simulink model "14_bus"  (R2024a)
settings: Solver=VariableStepAuto  StartTime=0.0  StopTime=1  RelTol=1e-3
undefined symbols (not defined in the file): D1, Delta
libraries: spsRMSLib x186, simulink_extras x171, spsThreePhaseVIMeasurementLib x94, spsThreePhaseBreakerLib x62, spsThreePhaseSeriesRLCBranchLib x20, spsThreePhaseSeriesRLCLoadLib x12, spsThreePhaseSourceLib x5, spsLoadFlowBusLib x5, spsStairGeneratorLib x5, spsThreePhaseTransformerTwoWindingsLib x5, spsThreePhaseFaultLib x5, sps_lib x1
(part 2 of 6)

== system 14_bus/BUS_3 ==
  Bus-3 : spsThreePhaseVIMeasurementLib/Three-Phase V-I Measurement  VoltageMeasurement=phase-to-ground  SetLabelV=on  LabelV=VB3  Vpu=off  VpuLL=off  CurrentMeasurement=yes  SetLabelI=on  LabelI=IB3  Ipu=off  Pbase=100e6  Vbase=0.95  OutputType=Complex  PhasorSimulation=off  PSBequivalent=0
  Bus3 : spsThreePhaseVIMeasurementLib/Three-Phase V-I Measurement  VoltageMeasurement=phase-to-ground  SetLabelV=on  LabelV=VB_3  Vpu=off  VpuLL=off  CurrentMeasurement=yes  SetLabelI=on  LabelI=IB_3  Ipu=off  Pbase=100e6  Vbase=0.95  OutputType=Complex  PhasorSimulation=off  PSBequivalent=0
  Bus_3 : spsThreePhaseVIMeasurementLib/Three-Phase V-I Measurement  VoltageMeasurement=phase-to-ground  SetLabelV=on  LabelV=V_B3  Vpu=off  VpuLL=off  CurrentMeasurement=yes  SetLabelI=on  LabelI=I_B3  Ipu=off  Pbase=100e6  Vbase=0.95  OutputType=Complex  PhasorSimulation=off  PSBequivalent=0
  C : PMIOPort  Side=Left
  B : PMIOPort  Port=2  Side=Left
  C1 : PMIOPort  Port=3  Side=Left
  c : PMIOPort  Port=4  Side=Right
  b : PMIOPort  Port=5  Side=Right
  a : PMIOPort  Port=6  Side=Right
  a1 : PMIOPort  Port=7  Side=Right
  b1 : PMIOPort  Port=8  Side=Right
  c1 : PMIOPort  Port=9  Side=Right
  a2 : PMIOPort  Port=10  Side=Right
  b2 : PMIOPort  Port=11  Side=Right
  c2 : PMIOPort  Port=12  Side=Right
  connections:
  b/RConn1 -- Bus-3/RConn2
  Bus_3/LConn3 -- Bus3/LConn1 -- C/RConn1 -- Bus-3/LConn3
  a/RConn1 -- Bus-3/RConn1
  c1/RConn1 -- Bus3/RConn3
  c/RConn1 -- Bus-3/RConn3
  Bus-3/LConn2 -- B/RConn1 -- Bus3/LConn2 -- Bus_3/LConn2
  Bus_3/LConn1 -- C1/RConn1 -- Bus-3/LConn1 -- Bus3/LConn3
  c2/RConn1 -- Bus_3/RConn3
  a1/RConn1 -- Bus3/RConn1
  b2/RConn1 -- Bus_3/RConn2
  b1/RConn1 -- Bus3/RConn2
  a2/RConn1 -- Bus_3/RConn1

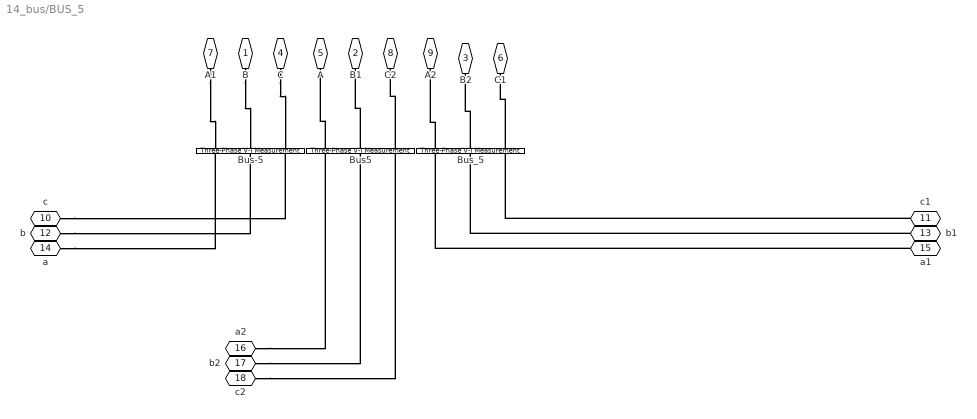
== system 14_bus/BUS_5 ==
  Bus-5 : spsThreePhaseVIMeasurementLib/Three-Phase V-I Measurement  VoltageMeasurement=phase-to-ground  SetLabelV=on  LabelV=VB5  Vpu=off  VpuLL=off  CurrentMeasurement=yes  SetLabelI=on  LabelI=IB5  Ipu=off  Pbase=100e6  Vbase=0.95  OutputType=Complex  PhasorSimulation=off  PSBequivalent=0
  Bus5 : spsThreePhaseVIMeasurementLib/Three-Phase V-I Measurement  VoltageMeasurement=phase-to-ground  SetLabelV=on  LabelV=VB_5  Vpu=off  VpuLL=off  CurrentMeasurement=yes  SetLabelI=on  LabelI=IB_5  Ipu=off  Pbase=100e6  Vbase=0.95  OutputType=Complex  PhasorSimulation=off  PSBequivalent=0
  Bus_5 : spsThreePhaseVIMeasurementLib/Three-Phase V-I Measurement  VoltageMeasurement=phase-to-ground  SetLabelV=on  LabelV=V_B5  Vpu=off  VpuLL=off  CurrentMeasurement=yes  SetLabelI=on  LabelI=I_B5  Ipu=off  Pbase=100e6  Vbase=0.95  OutputType=Complex  PhasorSimulation=off  PSBequivalent=0
  B : PMIOPort  Side=Left
  B1 : PMIOPort  Port=2  Side=Left
  B2 : PMIOPort  Port=3  Side=Left
  C : PMIOPort  Port=4  Side=Left
  A : PMIOPort  Port=5  Side=Left
  C1 : PMIOPort  Port=6  Side=Left
  A1 : PMIOPort  Port=7  Side=Left
  C2 : PMIOPort  Port=8  Side=Left
  A2 : PMIOPort  Port=9  Side=Left
  c : PMIOPort  Port=10  Side=Right
  c1 : PMIOPort  Port=11  Side=Right
  b : PMIOPort  Port=12  Side=Right
  b1 : PMIOPort  Port=13  Side=Right
  a : PMIOPort  Port=14  Side=Right
  a1 : PMIOPort  Port=15  Side=Right
  a2 : PMIOPort  Port=16  Side=Right
  b2 : PMIOPort  Port=17  Side=Right
  c2 : PMIOPort  Port=18  Side=Right
  connections:
  b/RConn1 -- Bus-5/RConn2
  c2/RConn1 -- Bus5/RConn3
  Bus5/LConn1 -- A/RConn1
  C/RConn1 -- Bus-5/LConn3
  Bus_5/LConn1 -- A2/RConn1
  c1/RConn1 -- Bus_5/RConn3
  B/RConn1 -- Bus-5/LConn2
  a1/RConn1 -- Bus_5/RConn1
  a2/RConn1 -- Bus5/RConn1
  Bus5/LConn2 -- B1/RConn1
  Bus_5/LConn2 -- B2/RConn1
  b1/RConn1 -- Bus_5/RConn2
  b2/RConn1 -- Bus5/RConn2
  c/RConn1 -- Bus-5/RConn3
  Bus5/LConn3 -- C2/RConn1
  A1/RConn1 -- Bus-5/LConn1
  Bus_5/LConn3 -- C1/RConn1
  a/RConn1 -- Bus-5/RConn1

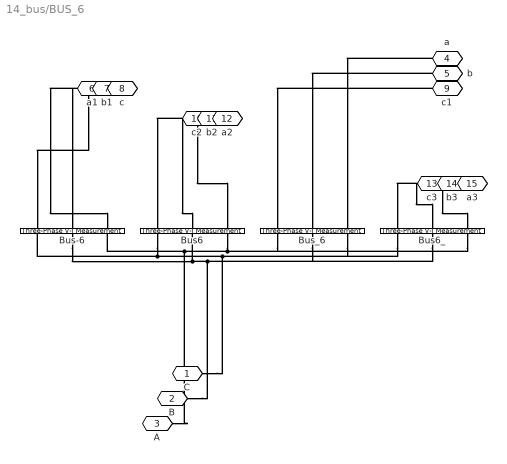
== system 14_bus/BUS_6 ==
  Bus-6 : spsThreePhaseVIMeasurementLib/Three-Phase V-I Measurement  VoltageMeasurement=phase-to-ground  SetLabelV=on  LabelV=VB6  Vpu=off  VpuLL=off  CurrentMeasurement=yes  SetLabelI=on  LabelI=IB6  Ipu=off  Pbase=100e6  Vbase=0.95  OutputType=Complex  PhasorSimulation=off  PSBequivalent=0
  Bus6 : spsThreePhaseVIMeasurementLib/Three-Phase V-I Measurement  VoltageMeasurement=phase-to-ground  SetLabelV=on  LabelV=VB_6  Vpu=off  VpuLL=off  CurrentMeasurement=yes  SetLabelI=on  LabelI=IB_6  Ipu=off  Pbase=100e6  Vbase=0.95  OutputType=Complex  PhasorSimulation=off  PSBequivalent=0
  Bus6_ : spsThreePhaseVIMeasurementLib/Three-Phase V-I Measurement  VoltageMeasurement=phase-to-ground  SetLabelV=on  LabelV=VB6_  Vpu=off  VpuLL=off  CurrentMeasurement=yes  SetLabelI=on  LabelI=IB6_  Ipu=off  Pbase=100e6  Vbase=0.95  OutputType=Complex  PhasorSimulation=off  PSBequivalent=0
  Bus_6 : spsThreePhaseVIMeasurementLib/Three-Phase V-I Measurement  VoltageMeasurement=phase-to-ground  SetLabelV=on  LabelV=V_B6  Vpu=off  VpuLL=off  CurrentMeasurement=yes  SetLabelI=on  LabelI=I_B6  Ipu=off  Pbase=100e6  Vbase=0.95  OutputType=Complex  PhasorSimulation=off  PSBequivalent=0
  C : PMIOPort  Side=Left
  B : PMIOPort  Port=2  Side=Left
  A : PMIOPort  Port=3  Side=Left
  a : PMIOPort  Port=4  Side=Right
  b : PMIOPort  Port=5  Side=Right
  a1 : PMIOPort  Port=6  Side=Right
  b1 : PMIOPort  Port=7  Side=Right
  c : PMIOPort  Port=8  Side=Right
  c1 : PMIOPort  Port=9  Side=Right
  c2 : PMIOPort  Port=10  Side=Right
  b2 : PMIOPort  Port=11  Side=Right
  a2 : PMIOPort  Port=12  Side=Right
  c3 : PMIOPort  Port=13  Side=Right
  b3 : PMIOPort  Port=14  Side=Right
  a3 : PMIOPort  Port=15  Side=Right
  connections:
  Bus6_/LConn1 -- Bus_6/LConn3 -- Bus6/LConn1 -- A/RConn1 -- Bus-6/LConn1
  b/RConn1 -- Bus_6/RConn2
  Bus6_/LConn3 -- Bus_6/LConn1 -- C/RConn1 -- Bus6/LConn3 -- Bus-6/LConn3
  c/RConn1 -- Bus-6/RConn3
  Bus6_/LConn2 -- Bus_6/LConn2 -- B/RConn1 -- Bus-6/LConn2 -- Bus6/LConn2
  a/RConn1 -- Bus_6/RConn1
  b1/RConn1 -- Bus-6/RConn2
  a3/RConn1 -- Bus6_/RConn1
  c1/RConn1 -- Bus_6/RConn3
  c3/RConn1 -- Bus6_/RConn3
  b3/RConn1 -- Bus6_/RConn2
  c2/RConn1 -- Bus6/RConn3
  a1/RConn1 -- Bus-6/RConn1
  a2/RConn1 -- Bus6/RConn1
  b2/RConn1 -- Bus6/RConn2

== system 14_bus/BUS_7 ==
  Bus-7 : spsThreePhaseVIMeasurementLib/Three-Phase V-I Measurement  VoltageMeasurement=phase-to-ground  SetLabelV=on  LabelV=VB7  Vpu=off  VpuLL=off  CurrentMeasurement=yes  SetLabelI=on  LabelI=IB7  Ipu=off  Pbase=100e6  Vbase=0.95  OutputType=Complex  PhasorSimulation=off  PSBequivalent=0
  Bus7 : spsThreePhaseVIMeasurementLib/Three-Phase V-I Measurement  VoltageMeasurement=phase-to-ground  SetLabelV=on  LabelV=VB_7  Vpu=off  VpuLL=off  CurrentMeasurement=yes  SetLabelI=on  LabelI=IB_7  Ipu=off  Pbase=100e6  Vbase=0.95  OutputType=Complex  PhasorSimulation=off  PSBequivalent=0
  a : PMIOPort  Side=Right
  b : PMIOPort  Port=2  Side=Right
  c : PMIOPort  Port=3  Side=Right
  a1 : PMIOPort  Port=4  Side=Right
  b1 : PMIOPort  Port=5  Side=Right
  c1 : PMIOPort  Port=6  Side=Right
  C : PMIOPort  Port=7  Side=Left
  B : PMIOPort  Port=8  Side=Left
  C1 : PMIOPort  Port=9  Side=Left
  connections:
  Bus7/LConn2 -- B/RConn1 -- Bus-7/LConn2
  Bus-7/LConn1 -- C/RConn1 -- Bus7/LConn3
  a1/RConn1 -- Bus7/RConn1
  Bus7/LConn1 -- Bus-7/LConn3 -- C1/RConn1
  b/RConn1 -- Bus-7/RConn2
  a/RConn1 -- Bus-7/RConn1
  b1/RConn1 -- Bus7/RConn2
  c1/RConn1 -- Bus7/RConn3
  c/RConn1 -- Bus-7/RConn3

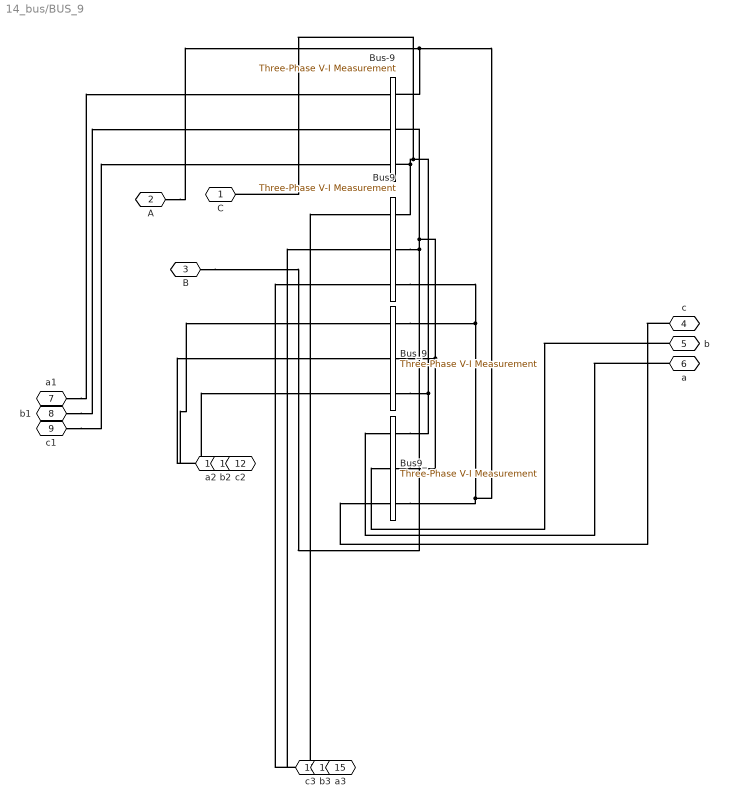
== system 14_bus/BUS_9 ==
  Bus-9 : spsThreePhaseVIMeasurementLib/Three-Phase V-I Measurement  VoltageMeasurement=phase-to-ground  SetLabelV=on  LabelV=VB9  Vpu=off  VpuLL=off  CurrentMeasurement=yes  SetLabelI=on  LabelI=IB9  Ipu=off  Pbase=100e6  Vbase=0.95  OutputType=Complex  PhasorSimulation=off  PSBequivalent=0
  Bus9 : spsThreePhaseVIMeasurementLib/Three-Phase V-I Measurement  VoltageMeasurement=phase-to-ground  SetLabelV=on  LabelV=VB_9  Vpu=off  VpuLL=off  CurrentMeasurement=yes  SetLabelI=on  LabelI=IB_9  Ipu=off  Pbase=100e6  Vbase=0.95  OutputType=Complex  PhasorSimulation=off  PSBequivalent=0
  Bus9_ : spsThreePhaseVIMeasurementLib/Three-Phase V-I Measurement  VoltageMeasurement=phase-to-ground  SetLabelV=on  LabelV=VB9_  Vpu=off  VpuLL=off  CurrentMeasurement=yes  SetLabelI=on  LabelI=IB9_  Ipu=off  Pbase=100e6  Vbase=0.95  OutputType=Complex  PhasorSimulation=off  PSBequivalent=0
  Bus_9 : spsThreePhaseVIMeasurementLib/Three-Phase V-I Measurement  VoltageMeasurement=phase-to-ground  SetLabelV=on  LabelV=V_B9  Vpu=off  VpuLL=off  CurrentMeasurement=yes  SetLabelI=on  LabelI=I_B9  Ipu=off  Pbase=100e6  Vbase=0.95  OutputType=Complex  PhasorSimulation=off  PSBequivalent=0
  C : PMIOPort  Side=Left
  A : PMIOPort  Port=2  Side=Left
  B : PMIOPort  Port=3  Side=Left
  c : PMIOPort  Port=4  Side=Right
  b : PMIOPort  Port=5  Side=Right
  a : PMIOPort  Port=6  Side=Right
  a1 : PMIOPort  Port=7  Side=Right
  b1 : PMIOPort  Port=8  Side=Right
  c1 : PMIOPort  Port=9  Side=Right
  a2 : PMIOPort  Port=10  Side=Right
  b2 : PMIOPort  Port=11  Side=Right
  c2 : PMIOPort  Port=12  Side=Right
  c3 : PMIOPort  Port=13  Side=Right
  b3 : PMIOPort  Port=14  Side=Right
  a3 : PMIOPort  Port=15  Side=Right
  connections:
  Bus9_/LConn1 -- Bus_9/LConn3 -- Bus9/LConn1 -- Bus-9/LConn3 -- C/RConn1
  A/RConn1 -- Bus-9/LConn1 -- Bus9_/LConn3 -- Bus9/LConn3 -- Bus_9/LConn1
  c/RConn1 -- Bus9_/RConn3
  B/RConn1 -- Bus9_/LConn2 -- Bus_9/LConn2 -- Bus-9/LConn2 -- Bus9/LConn2
  a3/RConn1 -- Bus9/RConn1
  c1/RConn1 -- Bus-9/RConn3
  b1/RConn1 -- Bus-9/RConn2
  c2/RConn1 -- Bus_9/RConn3
  a/RConn1 -- Bus9_/RConn1
  b2/RConn1 -- Bus_9/RConn2
  b/RConn1 -- Bus9_/RConn2
  b3/RConn1 -- Bus9/RConn2
  a2/RConn1 -- Bus_9/RConn1
  a1/RConn1 -- Bus-9/RConn1
  c3/RConn1 -- Bus9/RConn3

== system 14_bus/Subsystem1 ==
  Subsystem1 : Subsystem
  Three-Phase Breaker26 : spsThreePhaseBreakerLib/Three-Phase Breaker  InitialState=closed  SwitchA=on  SwitchB=on  SwitchC=on  SwitchTimes="[1/60  5/60]"  External=on  BreakerResistance=0.01  SnubberResistance=1e6  SnubberCapacitance=inf  Measurements=None
  VI13 : spsThreePhaseVIMeasurementLib/Three-Phase V-I Measurement  VoltageMeasurement=no  SetLabelV=off  LabelV=Vabc  Vpu=off  VpuLL=off  CurrentMeasurement=yes  SetLabelI=on  LabelI=I87  Ipu=off  Pbase=100e6  Vbase=500e3  OutputType=Complex  PhasorSimulation=off  PSBequivalent=0
  A : PMIOPort  Side=Left
  B : PMIOPort  Port=2  Side=Left
  C : PMIOPort  Port=3  Side=Left
  a : PMIOPort  Port=4  Side=Right
  b : PMIOPort  Port=5  Side=Right
  c : PMIOPort  Port=6  Side=Right
  wires:
  Subsystem1/1(Out1) -> Three-Phase Breaker26/1
  [I87] -> Subsystem1/1(Iabc1)
  connections:
  VI13/LConn1 -- A/RConn1
  Three-Phase Breaker26/LConn2 -- VI13/RConn2
  Three-Phase Breaker26/LConn3 -- VI13/RConn3
  Three-Phase Breaker26/LConn1 -- VI13/RConn1
  VI13/LConn2 -- B/RConn1
  Three-Phase Breaker26/RConn1 -- a/RConn1
  VI13/LConn3 -- C/RConn1
  Three-Phase Breaker26/RConn2 -- b/RConn1
  Three-Phase Breaker26/RConn3 -- c/RConn1

== system 14_bus/Subsystem10 ==
  Subsystem13 : Subsystem
  Three-Phase Breaker14 : spsThreePhaseBreakerLib/Three-Phase Breaker  InitialState=closed  SwitchA=on  SwitchB=on  SwitchC=on  SwitchTimes="[1/60  5/60]"  External=on  BreakerResistance=0.01  SnubberResistance=1e6  SnubberCapacitance=inf  Measurements=None
  VI5 : spsThreePhaseVIMeasurementLib/Three-Phase V-I Measurement  VoltageMeasurement=no  SetLabelV=off  LabelV=Vabc  Vpu=off  VpuLL=off  CurrentMeasurement=yes  SetLabelI=on  LabelI=I24  Ipu=off  Pbase=100e6  Vbase=500e3  OutputType=Complex  PhasorSimulation=off  PSBequivalent=0
  A : PMIOPort  Side=Left
  B : PMIOPort  Port=2  Side=Left
  a : PMIOPort  Port=3  Side=Right
  C : PMIOPort  Port=4  Side=Left
  b : PMIOPort  Port=5  Side=Right
  c : PMIOPort  Port=6  Side=Right
  wires:
  Subsystem13/1(Out1) -> Three-Phase Breaker14/1
  [I24] -> Subsystem13/1(Iabc1)
  connections:
  VI5/RConn2 -- b/RConn1
  Three-Phase Breaker14/LConn1 -- A/RConn1
  c/RConn1 -- VI5/RConn3
  VI5/LConn2 -- Three-Phase Breaker14/RConn2
  Three-Phase Breaker14/RConn1 -- VI5/LConn1
  Three-Phase Breaker14/RConn3 -- VI5/LConn3
  Three-Phase Breaker14/LConn2 -- B/RConn1
  a/RConn1 -- VI5/RConn1
  Three-Phase Breaker14/LConn3 -- C/RConn1

== system 14_bus/Subsystem11 ==
  Vabc : Inport
  Vabc1 : Inport  Port=2
  Subsystem12 : Subsystem
  Three-Phase Transformer (Two Windings)2 : spsThreePhaseTransformerTwoWindingsLib/Three-Phase Transformer (Two Windings)  Winding1Connection=Delta (D1)  Winding2Connection=Yg  CoreType=Three single-phase transformers  SetSaturation=off  Hysteresis=off  DataFile='hysteresis'  SetInitialFlux=off  Measurements=None  UNITS=pu  NominalPower=[ 250e6 , 50 ]  Winding1=[ 25e3*1.01 , 0.002 , 0.08 ]  Winding2=[ 25e3*1.01 , 0.002 , 0.08 ]  Rm=500  Lm=500  L0=0.5  Saturation=[ 0,0 ; 0.0024,1.2 ; 1.0,1.52 ]  InitialFluxes=[ 0.8 , -0.8 , 0.7 ]  BreakLoop=off  DiscreteSolver=Trapezoidal iterative  DataType=off  TransfoNumber=1
  Three-Phase Breaker12 : spsThreePhaseBreakerLib/Three-Phase Breaker  InitialState=closed  SwitchA=on  SwitchB=on  SwitchC=on  SwitchTimes="[1/60  5/60]"  External=on  BreakerResistance=0.01  SnubberResistance=1e6  SnubberCapacitance=inf  Measurements=None
  Three-Phase Breaker13 : spsThreePhaseBreakerLib/Three-Phase Breaker  InitialState=closed  SwitchA=on  SwitchB=on  SwitchC=on  SwitchTimes="[1/60  5/60]"  External=on  BreakerResistance=0.01  SnubberResistance=1e6  SnubberCapacitance=inf  Measurements=None
  c : PMIOPort  Side=Right
  b : PMIOPort  Port=2  Side=Right
  a : PMIOPort  Port=3  Side=Right
  C : PMIOPort  Port=4  Side=Left
  B : PMIOPort  Port=5  Side=Left
  A : PMIOPort  Port=6  Side=Left
  wires:
  Subsystem12/1(Out1) -> Three-Phase Breaker13/1, Three-Phase Breaker12/1
  Vabc1/1 -> Subsystem12/1(Vabc1)
  Vabc/1 -> Subsystem12/2(Vabc)
  connections:
  Three-Phase Breaker13/LConn2 -- Three-Phase Transformer (Two Windings)2/RConn2
  Three-Phase Breaker12/RConn3 -- Three-Phase Transformer (Two Windings)2/LConn3
  B/RConn1 -- Three-Phase Breaker12/LConn2
  Three-Phase Breaker12/RConn1 -- Three-Phase Transformer (Two Windings)2/LConn1
  Three-Phase Breaker12/RConn2 -- Three-Phase Transformer (Two Windings)2/LConn2
  Three-Phase Breaker13/RConn2 -- b/RConn1
  Three-Phase Breaker13/LConn3 -- Three-Phase Transformer (Two Windings)2/RConn3
  Three-Phase Breaker13/LConn1 -- Three-Phase Transformer (Two Windings)2/RConn1
  C/RConn1 -- Three-Phase Breaker12/LConn3
  Three-Phase Breaker13/RConn1 -- a/RConn1
  A/RConn1 -- Three-Phase Breaker12/LConn1
  Three-Phase Breaker13/RConn3 -- c/RConn1

== system 14_bus/Subsystem12 ==
  Subsystem1 : Subsystem
  Three-Phase Breaker26 : spsThreePhaseBreakerLib/Three-Phase Breaker  InitialState=closed  SwitchA=on  SwitchB=on  SwitchC=on  SwitchTimes="[1/60  5/60]"  External=on  BreakerResistance=0.01  SnubberResistance=1e6  SnubberCapacitance=inf  Measurements=None
  VI13 : spsThreePhaseVIMeasurementLib/Three-Phase V-I Measurement  VoltageMeasurement=no  SetLabelV=off  LabelV=Vabc  Vpu=off  VpuLL=off  CurrentMeasurement=yes  SetLabelI=on  LabelI=I34  Ipu=off  Pbase=100e6  Vbase=500e3  OutputType=Complex  PhasorSimulation=off  PSBequivalent=0
  A : PMIOPort  Side=Left
  B : PMIOPort  Port=2  Side=Left
  C : PMIOPort  Port=3  Side=Left
  a : PMIOPort  Port=4  Side=Right
  b : PMIOPort  Port=5  Side=Right
  c : PMIOPort  Port=6  Side=Right
  wires:
  Subsystem1/1(Out1) -> Three-Phase Breaker26/1
  [I34] -> Subsystem1/1(Iabc1)
  connections:
  VI13/LConn1 -- A/RConn1
  Three-Phase Breaker26/LConn2 -- VI13/RConn2
  Three-Phase Breaker26/LConn3 -- VI13/RConn3
  Three-Phase Breaker26/LConn1 -- VI13/RConn1
  VI13/LConn2 -- B/RConn1
  Three-Phase Breaker26/RConn1 -- a/RConn1
  VI13/LConn3 -- C/RConn1
  Three-Phase Breaker26/RConn2 -- b/RConn1
  Three-Phase Breaker26/RConn3 -- c/RConn1

== system 14_bus/Subsystem13 ==
  Subsystem1 : Subsystem
  Three-Phase Breaker26 : spsThreePhaseBreakerLib/Three-Phase Breaker  InitialState=closed  SwitchA=on  SwitchB=on  SwitchC=on  SwitchTimes="[1/60  5/60]"  External=on  BreakerResistance=0.01  SnubberResistance=1e6  SnubberCapacitance=inf  Measurements=None
  VI13 : spsThreePhaseVIMeasurementLib/Three-Phase V-I Measurement  VoltageMeasurement=no  SetLabelV=off  LabelV=Vabc  Vpu=off  VpuLL=off  CurrentMeasurement=yes  SetLabelI=on  LabelI=I42  Ipu=off  Pbase=100e6  Vbase=500e3  OutputType=Complex  PhasorSimulation=off  PSBequivalent=0
  A : PMIOPort  Side=Left
  B : PMIOPort  Port=2  Side=Left
  C : PMIOPort  Port=3  Side=Left
  a : PMIOPort  Port=4  Side=Right
  b : PMIOPort  Port=5  Side=Right
  c : PMIOPort  Port=6  Side=Right
  wires:
  Subsystem1/1(Out1) -> Three-Phase Breaker26/1
  [I42] -> Subsystem1/1(Iabc1)
  connections:
  VI13/LConn1 -- A/RConn1
  Three-Phase Breaker26/LConn2 -- VI13/RConn2
  Three-Phase Breaker26/LConn3 -- VI13/RConn3
  Three-Phase Breaker26/LConn1 -- VI13/RConn1
  VI13/LConn2 -- B/RConn1
  Three-Phase Breaker26/RConn1 -- a/RConn1
  VI13/LConn3 -- C/RConn1
  Three-Phase Breaker26/RConn2 -- b/RConn1
  Three-Phase Breaker26/RConn3 -- c/RConn1

== system 14_bus/Subsystem14 ==
  Subsystem22 : Subsystem
  Three-Phase Breaker23 : spsThreePhaseBreakerLib/Three-Phase Breaker  InitialState=closed  SwitchA=on  SwitchB=on  SwitchC=on  SwitchTimes="[1/60  5/60]"  External=on  BreakerResistance=0.01  SnubberResistance=1e6  SnubberCapacitance=inf  Measurements=None
  VI10 : spsThreePhaseVIMeasurementLib/Three-Phase V-I Measurement  VoltageMeasurement=no  SetLabelV=off  LabelV=Vabc  Vpu=off  VpuLL=off  CurrentMeasurement=yes  SetLabelI=on  LabelI=IL5  Ipu=off  Pbase=100e6  Vbase=500e3  OutputType=Complex  PhasorSimulation=off  PSBequivalent=0
  A : PMIOPort  Side=Left
  B : PMIOPort  Port=2  Side=Left
  C : PMIOPort  Port=3  Side=Left
  a : PMIOPort  Port=4  Side=Right
  b : PMIOPort  Port=5  Side=Right
  c : PMIOPort  Port=6  Side=Right
  wires:
  Subsystem22/1(Out1) -> Three-Phase Breaker23/1
  [IL5] -> Subsystem22/1(Iabc1)
  connections:
  VI10/RConn2 -- Three-Phase Breaker23/LConn2
  Three-Phase Breaker23/RConn3 -- c/RConn1
  Three-Phase Breaker23/RConn1 -- a/RConn1
  Three-Phase Breaker23/LConn1 -- VI10/RConn1
  VI10/RConn3 -- Three-Phase Breaker23/LConn3
  Three-Phase Breaker23/RConn2 -- b/RConn1
  VI10/LConn2 -- B/RConn1
  VI10/LConn3 -- C/RConn1
  A/RConn1 -- VI10/LConn1

== system 14_bus/Subsystem15 ==
  Subsystem8 : Subsystem
  Three-Phase Breaker8 : spsThreePhaseBreakerLib/Three-Phase Breaker  InitialState=closed  SwitchA=on  SwitchB=on  SwitchC=on  SwitchTimes="[1/60  5/60]"  External=on  BreakerResistance=0.01  SnubberResistance=1e6  SnubberCapacitance=inf  Measurements=None
  VI2 : spsThreePhaseVIMeasurementLib/Three-Phase V-I Measurement  VoltageMeasurement=no  SetLabelV=off  LabelV=Vabc  Vpu=off  VpuLL=off  CurrentMeasurement=yes  SetLabelI=on  LabelI=IL2  Ipu=off  Pbase=100e6  Vbase=500e3  OutputType=Complex  PhasorSimulation=off  PSBequivalent=0
  a : PMIOPort  Side=Right
  b : PMIOPort  Port=2  Side=Right
  c : PMIOPort  Port=3  Side=Right
  C : PMIOPort  Port=4  Side=Left
  B : PMIOPort  Port=5  Side=Left
  A : PMIOPort  Port=6  Side=Left
  wires:
  Subsystem8/1(Out1) -> Three-Phase Breaker8/1
  [IL2] -> Subsystem8/1(Iabc1)
  connections:
  Three-Phase Breaker8/LConn3 -- VI2/RConn3
  Three-Phase Breaker8/LConn1 -- VI2/RConn1
  VI2/LConn1 -- A/RConn1
  Three-Phase Breaker8/RConn1 -- a/RConn1
  Three-Phase Breaker8/LConn2 -- VI2/RConn2
  VI2/LConn3 -- C/RConn1
  Three-Phase Breaker8/RConn2 -- b/RConn1
  Three-Phase Breaker8/RConn3 -- c/RConn1
  VI2/LConn2 -- B/RConn1

== system 14_bus/Subsystem16 ==
  Subsystem15 : Subsystem
  Three-Phase Breaker16 : spsThreePhaseBreakerLib/Three-Phase Breaker  InitialState=closed  SwitchA=on  SwitchB=on  SwitchC=on  SwitchTimes="[1/60  5/60]"  External=on  BreakerResistance=0.01  SnubberResistance=1e6  SnubberCapacitance=inf  Measurements=None
  VI7 : spsThreePhaseVIMeasurementLib/Three-Phase V-I Measurement  VoltageMeasurement=no  SetLabelV=off  LabelV=Vabc  Vpu=off  VpuLL=off  CurrentMeasurement=yes  SetLabelI=on  LabelI=I25  Ipu=off  Pbase=100e6  Vbase=500e3  OutputType=Complex  PhasorSimulation=off  PSBequivalent=0
  a : PMIOPort  Side=Right
  b : PMIOPort  Port=2  Side=Right
  c : PMIOPort  Port=3  Side=Right
  A : PMIOPort  Port=4  Side=Left
  B : PMIOPort  Port=5  Side=Left
  C : PMIOPort  Port=6  Side=Left
  wires:
  Subsystem15/1(Out1) -> Three-Phase Breaker16/1
  [I25] -> Subsystem15/1(Iabc1)
  connections:
  VI7/LConn3 -- Three-Phase Breaker16/RConn3
  Three-Phase Breaker16/LConn3 -- C/RConn1
  VI7/LConn2 -- Three-Phase Breaker16/RConn2
  VI7/RConn2 -- b/RConn1
  Three-Phase Breaker16/LConn2 -- B/RConn1
  c/RConn1 -- VI7/RConn3
  VI7/LConn1 -- Three-Phase Breaker16/RConn1
  Three-Phase Breaker16/LConn1 -- A/RConn1
  a/RConn1 -- VI7/RConn1

== system 14_bus/Subsystem17 ==
  Subsystem1 : Subsystem
  Three-Phase Breaker26 : spsThreePhaseBreakerLib/Three-Phase Breaker  InitialState=closed  SwitchA=on  SwitchB=on  SwitchC=on  SwitchTimes="[1/60  5/60]"  External=on  BreakerResistance=0.01  SnubberResistance=1e6  SnubberCapacitance=inf  Measurements=None
  VI13 : spsThreePhaseVIMeasurementLib/Three-Phase V-I Measurement  VoltageMeasurement=no  SetLabelV=off  LabelV=Vabc  Vpu=off  VpuLL=off  CurrentMeasurement=yes  SetLabelI=on  LabelI=I45  Ipu=off  Pbase=100e6  Vbase=500e3  OutputType=Complex  PhasorSimulation=off  PSBequivalent=0
  A : PMIOPort  Side=Left
  B : PMIOPort  Port=2  Side=Left
  C : PMIOPort  Port=3  Side=Left
  a : PMIOPort  Port=4  Side=Right
  b : PMIOPort  Port=5  Side=Right
  c : PMIOPort  Port=6  Side=Right
  wires:
  Subsystem1/1(Out1) -> Three-Phase Breaker26/1
  [I45] -> Subsystem1/1(Iabc1)
  connections:
  VI13/LConn1 -- A/RConn1
  Three-Phase Breaker26/LConn2 -- VI13/RConn2
  Three-Phase Breaker26/LConn3 -- VI13/RConn3
  Three-Phase Breaker26/LConn1 -- VI13/RConn1
  VI13/LConn2 -- B/RConn1
  Three-Phase Breaker26/RConn1 -- a/RConn1
  VI13/LConn3 -- C/RConn1
  Three-Phase Breaker26/RConn2 -- b/RConn1
  Three-Phase Breaker26/RConn3 -- c/RConn1

== system 14_bus/Subsystem18 ==
  Subsystem1 : Subsystem
  Three-Phase Breaker26 : spsThreePhaseBreakerLib/Three-Phase Breaker  InitialState=closed  SwitchA=on  SwitchB=on  SwitchC=on  SwitchTimes="[1/60  5/60]"  External=on  BreakerResistance=0.01  SnubberResistance=1e6  SnubberCapacitance=inf  Measurements=None
  VI13 : spsThreePhaseVIMeasurementLib/Three-Phase V-I Measurement  VoltageMeasurement=no  SetLabelV=off  LabelV=Vabc  Vpu=off  VpuLL=off  CurrentMeasurement=yes  SetLabelI=on  LabelI=I23  Ipu=off  Pbase=100e6  Vbase=500e3  OutputType=Complex  PhasorSimulation=off  PSBequivalent=0
  A : PMIOPort  Side=Left
  B : PMIOPort  Port=2  Side=Left
  C : PMIOPort  Port=3  Side=Left
  a : PMIOPort  Port=4  Side=Right
  b : PMIOPort  Port=5  Side=Right
  c : PMIOPort  Port=6  Side=Right
  wires:
  Subsystem1/1(Out1) -> Three-Phase Breaker26/1
  [I23] -> Subsystem1/1(Iabc1)
  connections:
  VI13/LConn1 -- A/RConn1
  Three-Phase Breaker26/LConn2 -- VI13/RConn2
  Three-Phase Breaker26/LConn3 -- VI13/RConn3
  Three-Phase Breaker26/LConn1 -- VI13/RConn1
  VI13/LConn2 -- B/RConn1
  Three-Phase Breaker26/RConn1 -- a/RConn1
  VI13/LConn3 -- C/RConn1
  Three-Phase Breaker26/RConn2 -- b/RConn1
  Three-Phase Breaker26/RConn3 -- c/RConn1

== system 14_bus/Subsystem19 ==
  Subsystem21 : Subsystem
  Three-Phase Breaker22 : spsThreePhaseBreakerLib/Three-Phase Breaker  InitialState=closed  SwitchA=on  SwitchB=on  SwitchC=on  SwitchTimes="[1/60  5/60]"  External=on  BreakerResistance=0.01  SnubberResistance=1e6  SnubberCapacitance=inf  Measurements=None
  VI9 : spsThreePhaseVIMeasurementLib/Three-Phase V-I Measurement  VoltageMeasurement=no  SetLabelV=off  LabelV=Vabc  Vpu=off  VpuLL=off  CurrentMeasurement=yes  SetLabelI=on  LabelI=IL4  Ipu=off  Pbase=100e6  Vbase=500e3  OutputType=Complex  PhasorSimulation=off  PSBequivalent=0
  c : PMIOPort  Side=Right
  b : PMIOPort  Port=2  Side=Right
  a : PMIOPort  Port=3  Side=Right
  C : PMIOPort  Port=4  Side=Left
  B : PMIOPort  Port=5  Side=Left
  A : PMIOPort  Port=6  Side=Left
  wires:
  Subsystem21/1(Out1) -> Three-Phase Breaker22/1
  [IL4] -> Subsystem21/1(Iabc1)
  connections:
  VI9/RConn2 -- Three-Phase Breaker22/LConn2
  Three-Phase Breaker22/RConn3 -- c/RConn1
  B/RConn1 -- VI9/LConn2
  VI9/RConn3 -- Three-Phase Breaker22/LConn3
  Three-Phase Breaker22/LConn1 -- VI9/RConn1
  Three-Phase Breaker22/RConn1 -- a/RConn1
  C/RConn1 -- VI9/LConn3
  A/RConn1 -- VI9/LConn1
  Three-Phase Breaker22/RConn2 -- b/RConn1

== system 14_bus/Subsystem2 ==
  Subsystem1 : Subsystem
  Three-Phase Breaker26 : spsThreePhaseBreakerLib/Three-Phase Breaker  InitialState=closed  SwitchA=on  SwitchB=on  SwitchC=on  SwitchTimes="[1/60  5/60]"  External=on  BreakerResistance=0.01  SnubberResistance=1e6  SnubberCapacitance=inf  Measurements=None
  VI13 : spsThreePhaseVIMeasurementLib/Three-Phase V-I Measurement  VoltageMeasurement=no  SetLabelV=off  LabelV=Vabc  Vpu=off  VpuLL=off  CurrentMeasurement=yes  SetLabelI=on  LabelI=I51  Ipu=off  Pbase=100e6  Vbase=500e3  OutputType=Complex  PhasorSimulation=off  PSBequivalent=0
  A : PMIOPort  Side=Left
  B : PMIOPort  Port=2  Side=Left
  C : PMIOPort  Port=3  Side=Left
  a : PMIOPort  Port=4  Side=Right
  b : PMIOPort  Port=5  Side=Right
  c : PMIOPort  Port=6  Side=Right
  wires:
  Subsystem1/1(Out1) -> Three-Phase Breaker26/1
  [I51] -> Subsystem1/1(Iabc1)
  connections:
  VI13/LConn1 -- A/RConn1
  Three-Phase Breaker26/LConn2 -- VI13/RConn2
  Three-Phase Breaker26/LConn3 -- VI13/RConn3
  Three-Phase Breaker26/LConn1 -- VI13/RConn1
  VI13/LConn2 -- B/RConn1
  Three-Phase Breaker26/RConn1 -- a/RConn1
  VI13/LConn3 -- C/RConn1
  Three-Phase Breaker26/RConn2 -- b/RConn1
  Three-Phase Breaker26/RConn3 -- c/RConn1

== system 14_bus/Subsystem20 ==
  Subsystem1 : Subsystem
  Three-Phase Breaker26 : spsThreePhaseBreakerLib/Three-Phase Breaker  InitialState=closed  SwitchA=on  SwitchB=on  SwitchC=on  SwitchTimes="[1/60  5/60]"  External=on  BreakerResistance=0.01  SnubberResistance=1e6  SnubberCapacitance=inf  Measurements=None
  VI13 : spsThreePhaseVIMeasurementLib/Three-Phase V-I Measurement  VoltageMeasurement=no  SetLabelV=off  LabelV=Vabc  Vpu=off  VpuLL=off  CurrentMeasurement=yes  SetLabelI=on  LabelI=I43  Ipu=off  Pbase=100e6  Vbase=500e3  OutputType=Complex  PhasorSimulation=off  PSBequivalent=0
  A : PMIOPort  Side=Left
  B : PMIOPort  Port=2  Side=Left
  C : PMIOPort  Port=3  Side=Left
  a : PMIOPort  Port=4  Side=Right
  b : PMIOPort  Port=5  Side=Right
  c : PMIOPort  Port=6  Side=Right
  wires:
  Subsystem1/1(Out1) -> Three-Phase Breaker26/1
  [I43] -> Subsystem1/1(Iabc1)
  connections:
  VI13/LConn1 -- A/RConn1
  Three-Phase Breaker26/LConn2 -- VI13/RConn2
  Three-Phase Breaker26/LConn3 -- VI13/RConn3
  Three-Phase Breaker26/LConn1 -- VI13/RConn1
  VI13/LConn2 -- B/RConn1
  Three-Phase Breaker26/RConn1 -- a/RConn1
  VI13/LConn3 -- C/RConn1
  Three-Phase Breaker26/RConn2 -- b/RConn1
  Three-Phase Breaker26/RConn3 -- c/RConn1

== system 14_bus/Subsystem21 ==
  Subsystem23 : Subsystem
  Three-Phase Breaker24 : spsThreePhaseBreakerLib/Three-Phase Breaker  InitialState=closed  SwitchA=on  SwitchB=on  SwitchC=on  SwitchTimes="[1/60  5/60]"  External=on  BreakerResistance=0.01  SnubberResistance=1e6  SnubberCapacitance=inf  Measurements=None
  VI11 : spsThreePhaseVIMeasurementLib/Three-Phase V-I Measurement  VoltageMeasurement=no  SetLabelV=off  LabelV=Vabc  Vpu=off  VpuLL=off  CurrentMeasurement=yes  SetLabelI=on  LabelI=I49  Ipu=off  Pbase=100e6  Vbase=500e3  OutputType=Complex  PhasorSimulation=off  PSBequivalent=0
  A : PMIOPort  Side=Left
  B : PMIOPort  Port=2  Side=Left
  C : PMIOPort  Port=3  Side=Left
  c : PMIOPort  Port=4  Side=Right
  b : PMIOPort  Port=5  Side=Right
  a : PMIOPort  Port=6  Side=Right
  wires:
  Subsystem23/1(Out1) -> Three-Phase Breaker24/1
  [I49] -> Subsystem23/1(Iabc1)
  connections:
  Three-Phase Breaker24/LConn1 -- VI11/RConn1
  Three-Phase Breaker24/LConn2 -- VI11/RConn2
  Three-Phase Breaker24/LConn3 -- VI11/RConn3
  Three-Phase Breaker24/RConn1 -- a/RConn1
  VI11/LConn2 -- B/RConn1
  Three-Phase Breaker24/RConn3 -- c/RConn1
  Three-Phase Breaker24/RConn2 -- b/RConn1
  C/RConn1 -- VI11/LConn3
  A/RConn1 -- VI11/LConn1

== system 14_bus/Subsystem22 ==
  Subsystem1 : Subsystem
  Three-Phase Breaker26 : spsThreePhaseBreakerLib/Three-Phase Breaker  InitialState=closed  SwitchA=on  SwitchB=on  SwitchC=on  SwitchTimes="[1/60  5/60]"  External=on  BreakerResistance=0.01  SnubberResistance=1e6  SnubberCapacitance=inf  Measurements=None
  VI13 : spsThreePhaseVIMeasurementLib/Three-Phase V-I Measurement  VoltageMeasurement=no  SetLabelV=off  LabelV=Vabc  Vpu=off  VpuLL=off  CurrentMeasurement=yes  SetLabelI=on  LabelI=I15  Ipu=off  Pbase=100e6  Vbase=500e3  OutputType=Complex  PhasorSimulation=off  PSBequivalent=0
  A : PMIOPort  Side=Left
  B : PMIOPort  Port=2  Side=Left
  C : PMIOPort  Port=3  Side=Left
  a : PMIOPort  Port=4  Side=Right
  b : PMIOPort  Port=5  Side=Right
  c : PMIOPort  Port=6  Side=Right
  wires:
  Subsystem1/1(Out1) -> Three-Phase Breaker26/1
  [I15] -> Subsystem1/1(Iabc1)
  connections:
  VI13/LConn1 -- A/RConn1
  Three-Phase Breaker26/LConn2 -- VI13/RConn2
  Three-Phase Breaker26/LConn3 -- VI13/RConn3
  Three-Phase Breaker26/LConn1 -- VI13/RConn1
  VI13/LConn2 -- B/RConn1
  Three-Phase Breaker26/RConn1 -- a/RConn1
  VI13/LConn3 -- C/RConn1
  Three-Phase Breaker26/RConn2 -- b/RConn1
  Three-Phase Breaker26/RConn3 -- c/RConn1

== system 14_bus/Subsystem23 ==
  Subsystem24 : Subsystem
      settings: PortSchema="{\"entries\":[{\"content\":{\"sides\":[{\"content\":{},\"type\":\"ConnectorPlacement.EquallySpacedRectSide\",\"uuid\":\"58e6417c-fd42-45d0-8699-7f185c6e0046\"},{\"content\":{\"connectorIds\":[\"Out1\"],\"side\":\"RIGHT\"},\"type\":\"ConnectorPlacement.EquallySpacedRectSide\",\"uuid\":\"611e248e-e50c-4541-8696-b11da3366a52\"},{\"content\":{\"side\":\"TOP\"},\"type\":\"ConnectorPlacement.EquallySpacedRectSide\",\"uuid\":\"8ad030e9-8f6f-4bf8-b510-47d84f85bf62\"},{\"content\":{\"connectorIds\":[\"In1\"],\"side\":\"BOTTOM\"},\"type\":\"ConnectorPlacement.EquallySpacedRectSide\",\"uuid\":\"0a68c041-45ac-4353-af8e-20296580d9e1\"}]},\"type\":\"ConnectorPlacement.EquallySpacedConnector\",\"uuid\":\"ccad7e75-59a4-4fa5-abd8-5d887d393a17\"}],\"packageUris\":[\"http://schema.mathworks.com/mf0/Connector/R2020b\"],\"version\":\"1.0\"}"
  Three-Phase Breaker25 : spsThreePhaseBreakerLib/Three-Phase Breaker  InitialState=closed  SwitchA=on  SwitchB=on  SwitchC=on  SwitchTimes="[1/60  5/60]"  External=on  BreakerResistance=0.01  SnubberResistance=1e6  SnubberCapacitance=inf  Measurements=None
  VI12 : spsThreePhaseVIMeasurementLib/Three-Phase V-I Measurement  VoltageMeasurement=no  SetLabelV=off  LabelV=Vabc  Vpu=off  VpuLL=off  CurrentMeasurement=yes  SetLabelI=on  LabelI=I94  Ipu=off  Pbase=100e6  Vbase=500e3  OutputType=Complex  PhasorSimulation=off  PSBequivalent=0
  A : PMIOPort  Side=Left
  B : PMIOPort  Port=2  Side=Left
  C : PMIOPort  Port=3  Side=Left
  a : PMIOPort  Port=4  Side=Right
  b : PMIOPort  Port=5  Side=Right
  c : PMIOPort  Port=6  Side=Right
  wires:
  Subsystem24/1(Out1) -> Three-Phase Breaker25/1
  [I94] -> Subsystem24/1(Iabc1)
  connections:
  VI12/LConn1 -- A/RConn1
  Three-Phase Breaker25/LConn3 -- VI12/RConn3
  Three-Phase Breaker25/LConn1 -- VI12/RConn1
  Three-Phase Breaker25/LConn2 -- VI12/RConn2
  Three-Phase Breaker25/RConn2 -- b/RConn1
  Three-Phase Breaker25/RConn3 -- c/RConn1
  VI12/LConn2 -- B/RConn1
  VI12/LConn3 -- C/RConn1
  Three-Phase Breaker25/RConn1 -- a/RConn1

== system 14_bus/Subsystem25 ==
  Vabc : Inport
  In2 : Inport  Port=2
  Subsystem27 : Subsystem
  Three-Phase Transformer (Two Windings)4 : spsThreePhaseTransformerTwoWindingsLib/Three-Phase Transformer (Two Windings)  Winding1Connection=Delta (D1)  Winding2Connection=Yg  CoreType=Three single-phase transformers  SetSaturation=off  Hysteresis=off  DataFile='hysteresis'  SetInitialFlux=off  Measurements=None  UNITS=pu  NominalPower=[ 250e6 , 50 ]  Winding1=[ 25e3*1.09 , 0.002 , 0.08 ]  Winding2=[ 25e3*1.09 , 0.002 , 0.08 ]  Rm=500  Lm=500  L0=0.5  Saturation=[ 0,0 ; 0.0024,1.2 ; 1.0,1.52 ]  InitialFluxes=[ 0.8 , -0.8 , 0.7 ]  BreakLoop=off  DiscreteSolver=Trapezoidal iterative  DataType=off  TransfoNumber=1
  Three-Phase Breaker28 : spsThreePhaseBreakerLib/Three-Phase Breaker  InitialState=closed  SwitchA=on  SwitchB=on  SwitchC=on  SwitchTimes="[1/60  5/60]"  External=on  BreakerResistance=0.01  SnubberResistance=1e6  SnubberCapacitance=inf  Measurements=None
  Three-Phase Breaker29 : spsThreePhaseBreakerLib/Three-Phase Breaker  InitialState=closed  SwitchA=on  SwitchB=on  SwitchC=on  SwitchTimes="[1/60  5/60]"  External=on  BreakerResistance=0.01  SnubberResistance=1e6  SnubberCapacitance=inf  Measurements=None
  a : PMIOPort  Side=Right
  b : PMIOPort  Port=2  Side=Right
  c : PMIOPort  Port=3  Side=Right
  A : PMIOPort  Port=4  Side=Left
  B : PMIOPort  Port=5  Side=Left
  C : PMIOPort  Port=6  Side=Left
  wires:
  Subsystem27/1(Out1) -> Three-Phase Breaker28/1, Three-Phase Breaker29/1
  Vabc/1 -> Subsystem27/2(Vabc)
  In2/1 -> Subsystem27/1(In1)
  connections:
  Three-Phase Transformer (Two Windings)4/LConn2 -- Three-Phase Breaker29/RConn2
  Three-Phase Breaker28/LConn3 -- Three-Phase Transformer (Two Windings)4/RConn3
  Three-Phase Transformer (Two Windings)4/LConn3 -- Three-Phase Breaker29/RConn3
  Three-Phase Breaker28/LConn2 -- Three-Phase Transformer (Two Windings)4/RConn2
  Three-Phase Breaker28/LConn1 -- Three-Phase Transformer (Two Windings)4/RConn1
  Three-Phase Transformer (Two Windings)4/LConn1 -- Three-Phase Breaker29/RConn1
  Three-Phase Breaker28/RConn2 -- b/RConn1
  Three-Phase Breaker28/RConn1 -- a/RConn1
  Three-Phase Breaker29/LConn1 -- A/RConn1
  Three-Phase Breaker28/RConn3 -- c/RConn1
  Three-Phase Breaker29/LConn3 -- C/RConn1
  Three-Phase Breaker29/LConn2 -- B/RConn1

== system 14_bus/Subsystem26 ==
  Subsystem25 : Subsystem
  Three-Phase Breaker26 : spsThreePhaseBreakerLib/Three-Phase Breaker  InitialState=closed  SwitchA=on  SwitchB=on  SwitchC=on  SwitchTimes="[1/60  5/60]"  External=on  BreakerResistance=0.01  SnubberResistance=1e6  SnubberCapacitance=inf  Measurements=None
  VI13 : spsThreePhaseVIMeasurementLib/Three-Phase V-I Measurement  VoltageMeasurement=no  SetLabelV=off  LabelV=Vabc  Vpu=off  VpuLL=off  CurrentMeasurement=yes  SetLabelI=on  LabelI=I47  Ipu=off  Pbase=100e6  Vbase=500e3  OutputType=Complex  PhasorSimulation=off  PSBequivalent=0
  A : PMIOPort  Side=Left
  B : PMIOPort  Port=2  Side=Left
  C : PMIOPort  Port=3  Side=Left
  c : PMIOPort  Port=4  Side=Right
  b : PMIOPort  Port=5  Side=Right
  a : PMIOPort  Port=6  Side=Right
  wires:
  Subsystem25/1(Out1) -> Three-Phase Breaker26/1
  [I47] -> Subsystem25/1(Iabc1)
  connections:
  VI13/LConn3 -- C/RConn1
  Three-Phase Breaker26/LConn3 -- VI13/RConn3
  Three-Phase Breaker26/RConn2 -- b/RConn1
  VI13/LConn1 -- A/RConn1
  Three-Phase Breaker26/RConn1 -- a/RConn1
  Three-Phase Breaker26/LConn1 -- VI13/RConn1
  Three-Phase Breaker26/LConn2 -- VI13/RConn2
  Three-Phase Breaker26/RConn3 -- c/RConn1
  VI13/LConn2 -- B/RConn1

== system 14_bus/Subsystem27 ==
  In1 : Inport
  Vabc : Inport  Port=2
  Scope : Scope
  Subsystem1 : Subsystem
  Three-Phase Transformer (Two Windings) : spsThreePhaseTransformerTwoWindingsLib/Three-Phase Transformer (Two Windings)  Winding1Connection=Delta (D1)  Winding2Connection=Yg  CoreType=Three single-phase transformers  SetSaturation=off  Hysteresis=off  DataFile='hysteresis'  SetInitialFlux=off  Measurements=None  UNITS=pu  NominalPower=[ 250e6 , 50 ]  Winding1=[ 25e3*1.060 , 0.002 , 0.08 ]  Winding2=[ 25e3*1.060 , 0.002 , 0.08 ]  Rm=500  Lm=500  L0=0.5  Saturation=[ 0,0 ; 0.0024,1.2 ; 1.0,1.52 ]  InitialFluxes=[ 0.8 , -0.8 , 0.7 ]  BreakLoop=off  DiscreteSolver=Trapezoidal iterative  DataType=off  TransfoNumber=1
  Three-Phase Breaker : spsThreePhaseBreakerLib/Three-Phase Breaker  InitialState=closed  SwitchA=on  SwitchB=on  SwitchC=on  SwitchTimes="[1/60  5/60]"  External=on  BreakerResistance=0.01  SnubberResistance=1e6  SnubberCapacitance=inf  Measurements=None
  Three-Phase Breaker1 : spsThreePhaseBreakerLib/Three-Phase Breaker  InitialState=closed  SwitchA=on  SwitchB=on  SwitchC=on  SwitchTimes="[1/60  5/60]"  External=on  BreakerResistance=0.01  SnubberResistance=1e6  SnubberCapacitance=inf  Measurements=None
  A : PMIOPort  Side=Left
  B : PMIOPort  Port=2  Side=Left
  C : PMIOPort  Port=3  Side=Left
  a : PMIOPort  Port=4  Side=Right
  b : PMIOPort  Port=5  Side=Right
  c : PMIOPort  Port=6  Side=Right
  wires:
  Vabc/1 -> Subsystem1/2(Vabc)
  Subsystem1/1(Out1) -> Scope/1, Three-Phase Breaker1/1, Three-Phase Breaker/1
  In1/1 -> Subsystem1/1(In1)
  connections:
  C/RConn1 -- Three-Phase Breaker/LConn3
  A/RConn1 -- Three-Phase Breaker/LConn1
  Three-Phase Breaker1/LConn2 -- Three-Phase Transformer (Two Windings)/RConn2
  Three-Phase Breaker/RConn1 -- Three-Phase Transformer (Two Windings)/LConn1
  Three-Phase Breaker/RConn3 -- Three-Phase Transformer (Two Windings)/LConn3
  Three-Phase Breaker1/LConn1 -- Three-Phase Transformer (Two Windings)/RConn1
  Three-Phase Breaker/RConn2 -- Three-Phase Transformer (Two Windings)/LConn2
  Three-Phase Breaker1/LConn3 -- Three-Phase Transformer (Two Windings)/RConn3
  Three-Phase Breaker1/RConn3 -- c/RConn1
  Three-Phase Breaker1/RConn1 -- a/RConn1
  B/RConn1 -- Three-Phase Breaker/LConn2
  Three-Phase Breaker1/RConn2 -- b/RConn1

== system 14_bus/Subsystem28 ==
  Subsystem1 : Subsystem
  Three-Phase Breaker26 : spsThreePhaseBreakerLib/Three-Phase Breaker  InitialState=closed  SwitchA=on  SwitchB=on  SwitchC=on  SwitchTimes="[1/60  5/60]"  External=on  BreakerResistance=0.01  SnubberResistance=1e6  SnubberCapacitance=inf  Measurements=None
  VI13 : spsThreePhaseVIMeasurementLib/Three-Phase V-I Measurement  VoltageMeasurement=no  SetLabelV=off  LabelV=Vabc  Vpu=off  VpuLL=off  CurrentMeasurement=yes  SetLabelI=on  LabelI=I54  Ipu=off  Pbase=100e6  Vbase=500e3  OutputType=Complex  PhasorSimulation=off  PSBequivalent=0
  A : PMIOPort  Side=Left
  B : PMIOPort  Port=2  Side=Left
  C : PMIOPort  Port=3  Side=Left
  a : PMIOPort  Port=4  Side=Right
  b : PMIOPort  Port=5  Side=Right
  c : PMIOPort  Port=6  Side=Right
  wires:
  Subsystem1/1(Out1) -> Three-Phase Breaker26/1
  [I54] -> Subsystem1/1(Iabc1)
  connections:
  VI13/LConn1 -- A/RConn1
  Three-Phase Breaker26/LConn2 -- VI13/RConn2
  Three-Phase Breaker26/LConn3 -- VI13/RConn3
  Three-Phase Breaker26/LConn1 -- VI13/RConn1
  VI13/LConn2 -- B/RConn1
  Three-Phase Breaker26/RConn1 -- a/RConn1
  VI13/LConn3 -- C/RConn1
  Three-Phase Breaker26/RConn2 -- b/RConn1
  Three-Phase Breaker26/RConn3 -- c/RConn1

== system 14_bus/Subsystem29 ==
  Vabc : Inport
  In1 : Inport  Port=2
  Subsystem1 : Subsystem
  Three-Phase Transformer (Two Windings)3 : spsThreePhaseTransformerTwoWindingsLib/Three-Phase Transformer (Two Windings)  Winding1Connection=Delta (D1)  Winding2Connection=Yg  CoreType=Three single-phase transformers  SetSaturation=off  Hysteresis=off  DataFile='hysteresis'  SetInitialFlux=off  Measurements=None  UNITS=pu  NominalPower=[ 250e6 , 50 ]  Winding1=[ 25e3*1.07 , 0.002 , 0.08 ]  Winding2=[ 25e3*1.07 , 0.002 , 0.08 ]  Rm=500  Lm=500  L0=0.5  Saturation=[ 0,0 ; 0.0024,1.2 ; 1.0,1.52 ]  InitialFluxes=[ 0.8 , -0.8 , 0.7 ]  BreakLoop=off  DiscreteSolver=Trapezoidal iterative  DataType=off  TransfoNumber=1
  Three-Phase Breaker : spsThreePhaseBreakerLib/Three-Phase Breaker  InitialState=closed  SwitchA=on  SwitchB=on  SwitchC=on  SwitchTimes="[1/60  5/60]"  External=on  BreakerResistance=0.01  SnubberResistance=1e6  SnubberCapacitance=inf  Measurements=None
  Three-Phase Breaker1 : spsThreePhaseBreakerLib/Three-Phase Breaker  InitialState=closed  SwitchA=on  SwitchB=on  SwitchC=on  SwitchTimes="[1/60  5/60]"  External=on  BreakerResistance=0.01  SnubberResistance=1e6  SnubberCapacitance=inf  Measurements=None
  A : PMIOPort  Side=Left
  B : PMIOPort  Port=2  Side=Left
  C : PMIOPort  Port=3  Side=Left
  a : PMIOPort  Port=4  Side=Right
  b : PMIOPort  Port=5  Side=Right
  c : PMIOPort  Port=6  Side=Right
  wires:
  Vabc/1 -> Subsystem1/2(Vabc)
  Subsystem1/1(Out1) -> Three-Phase Breaker1/1, Three-Phase Breaker/1
  In1/1 -> Subsystem1/1(In1)
  connections:
  C/RConn1 -- Three-Phase Breaker/LConn3
  A/RConn1 -- Three-Phase Breaker/LConn1
  Three-Phase Transformer (Two Windings)3/RConn2 -- Three-Phase Breaker1/LConn2
  Three-Phase Transformer (Two Windings)3/LConn1 -- Three-Phase Breaker/RConn1
  Three-Phase Transformer (Two Windings)3/LConn3 -- Three-Phase Breaker/RConn3
  Three-Phase Transformer (Two Windings)3/RConn1 -- Three-Phase Breaker1/LConn1
  Three-Phase Transformer (Two Windings)3/LConn2 -- Three-Phase Breaker/RConn2
  Three-Phase Transformer (Two Windings)3/RConn3 -- Three-Phase Breaker1/LConn3
  Three-Phase Breaker1/RConn3 -- c/RConn1
  Three-Phase Breaker1/RConn1 -- a/RConn1
  B/RConn1 -- Three-Phase Breaker/LConn2
  Three-Phase Breaker1/RConn2 -- b/RConn1

== system 14_bus/Subsystem3 ==
  Subsystem16 : Subsystem
      settings: PortSchema="{\"entries\":[{\"content\":{\"sides\":[{\"content\":{},\"type\":\"ConnectorPlacement.EquallySpacedRectSide\",\"uuid\":\"58e6417c-fd42-45d0-8699-7f185c6e0046\"},{\"content\":{\"connectorIds\":[\"Out1\"],\"side\":\"RIGHT\"},\"type\":\"ConnectorPlacement.EquallySpacedRectSide\",\"uuid\":\"611e248e-e50c-4541-8696-b11da3366a52\"},{\"content\":{\"connectorIds\":[\"In1\"],\"side\":\"TOP\"},\"type\":\"ConnectorPlacement.EquallySpacedRectSide\",\"uuid\":\"8ad030e9-8f6f-4bf8-b510-47d84f85bf62\"}]},\"type\":\"ConnectorPlacement.EquallySpacedConnector\",\"uuid\":\"ccad7e75-59a4-4fa5-abd8-5d887d393a17\"}],\"packageUris\":[\"http://schema.mathworks.com/mf0/Connector/R2020b\"],\"version\":\"1.0\"}"
  Three-Phase Breaker17 : spsThreePhaseBreakerLib/Three-Phase Breaker  InitialState=closed  SwitchA=on  SwitchB=on  SwitchC=on  SwitchTimes="[1/60  5/60]"  External=on  BreakerResistance=0.01  SnubberResistance=1e6  SnubberCapacitance=inf  Measurements=None
  VI8 : spsThreePhaseVIMeasurementLib/Three-Phase V-I Measurement  VoltageMeasurement=no  SetLabelV=off  LabelV=Vabc  Vpu=off  VpuLL=off  CurrentMeasurement=yes  SetLabelI=on  LabelI=I52  Ipu=off  Pbase=100e6  Vbase=500e3  OutputType=Complex  PhasorSimulation=off  PSBequivalent=0
  a : PMIOPort  Side=Right
  b : PMIOPort  Port=2  Side=Right
  c : PMIOPort  Port=3  Side=Right
  A : PMIOPort  Port=4  Side=Left
  B : PMIOPort  Port=5  Side=Left
  C : PMIOPort  Port=6  Side=Left
  wires:
  Subsystem16/1(Out1) -> Three-Phase Breaker17/1
  [I52] -> Subsystem16/1(Iabc1)
  connections:
  C/RConn1 -- VI8/LConn3
  Three-Phase Breaker17/LConn3 -- VI8/RConn3
  Three-Phase Breaker17/RConn2 -- b/RConn1
  Three-Phase Breaker17/LConn1 -- VI8/RConn1
  Three-Phase Breaker17/LConn2 -- VI8/RConn2
  B/RConn1 -- VI8/LConn2
  Three-Phase Breaker17/RConn1 -- a/RConn1
  A/RConn1 -- VI8/LConn1
  Three-Phase Breaker17/RConn3 -- c/RConn1

== system 14_bus/Subsystem30 ==
  Subsystem1 : Subsystem
  Three-Phase Breaker26 : spsThreePhaseBreakerLib/Three-Phase Breaker  InitialState=closed  SwitchA=on  SwitchB=on  SwitchC=on  SwitchTimes="[1/60  5/60]"  External=on  BreakerResistance=0.01  SnubberResistance=1e6  SnubberCapacitance=inf  Measurements=None
  VI13 : spsThreePhaseVIMeasurementLib/Three-Phase V-I Measurement  VoltageMeasurement=no  SetLabelV=off  LabelV=Vabc  Vpu=off  VpuLL=off  CurrentMeasurement=yes  SetLabelI=on  LabelI=I78  Ipu=off  Pbase=100e6  Vbase=500e3  OutputType=Complex  PhasorSimulation=off  PSBequivalent=0
  A : PMIOPort  Side=Left
  B : PMIOPort  Port=2  Side=Left
  C : PMIOPort  Port=3  Side=Left
  a : PMIOPort  Port=4  Side=Right
  b : PMIOPort  Port=5  Side=Right
  c : PMIOPort  Port=6  Side=Right
  wires:
  Subsystem1/1(Out1) -> Three-Phase Breaker26/1
  [I78] -> Subsystem1/1(Iabc1)
  connections:
  VI13/LConn1 -- A/RConn1
  Three-Phase Breaker26/LConn2 -- VI13/RConn2
  Three-Phase Breaker26/LConn3 -- VI13/RConn3
  Three-Phase Breaker26/LConn1 -- VI13/RConn1
  VI13/LConn2 -- B/RConn1
  Three-Phase Breaker26/RConn1 -- a/RConn1
  VI13/LConn3 -- C/RConn1
  Three-Phase Breaker26/RConn2 -- b/RConn1
  Three-Phase Breaker26/RConn3 -- c/RConn1

== system 14_bus/Subsystem31 ==
  Subsystem1 : Subsystem
  Three-Phase Breaker26 : spsThreePhaseBreakerLib/Three-Phase Breaker  InitialState=closed  SwitchA=on  SwitchB=on  SwitchC=on  SwitchTimes="[1/60  5/60]"  External=on  BreakerResistance=0.01  SnubberResistance=1e6  SnubberCapacitance=inf  Measurements=None
  VI13 : spsThreePhaseVIMeasurementLib/Three-Phase V-I Measurement  VoltageMeasurement=no  SetLabelV=off  LabelV=Vabc  Vpu=off  VpuLL=off  CurrentMeasurement=yes  SetLabelI=on  LabelI=I79  Ipu=off  Pbase=100e6  Vbase=500e3  OutputType=Complex  PhasorSimulation=off  PSBequivalent=0
  A : PMIOPort  Side=Left
  B : PMIOPort  Port=2  Side=Left
  C : PMIOPort  Port=3  Side=Left
  a : PMIOPort  Port=4  Side=Right
  b : PMIOPort  Port=5  Side=Right
  c : PMIOPort  Port=6  Side=Right
  wires:
  Subsystem1/1(Out1) -> Three-Phase Breaker26/1
  [I79] -> Subsystem1/1(Iabc1)
  connections:
  VI13/LConn1 -- A/RConn1
  Three-Phase Breaker26/LConn2 -- VI13/RConn2
  Three-Phase Breaker26/LConn3 -- VI13/RConn3
  Three-Phase Breaker26/LConn1 -- VI13/RConn1
  VI13/LConn2 -- B/RConn1
  Three-Phase Breaker26/RConn1 -- a/RConn1
  VI13/LConn3 -- C/RConn1
  Three-Phase Breaker26/RConn2 -- b/RConn1
  Three-Phase Breaker26/RConn3 -- c/RConn1

== system 14_bus/Subsystem32 ==
  Subsystem1 : Subsystem
  Three-Phase Breaker26 : spsThreePhaseBreakerLib/Three-Phase Breaker  InitialState=closed  SwitchA=on  SwitchB=on  SwitchC=on  SwitchTimes="[1/60  5/60]"  External=on  BreakerResistance=0.01  SnubberResistance=1e6  SnubberCapacitance=inf  Measurements=None
  VI13 : spsThreePhaseVIMeasurementLib/Three-Phase V-I Measurement  VoltageMeasurement=no  SetLabelV=off  LabelV=Vabc  Vpu=off  VpuLL=off  CurrentMeasurement=yes  SetLabelI=on  LabelI=I97  Ipu=off  Pbase=100e6  Vbase=500e3  OutputType=Complex  PhasorSimulation=off  PSBequivalent=0
  A : PMIOPort  Side=Left
  B : PMIOPort  Port=2  Side=Left
  C : PMIOPort  Port=3  Side=Left
  a : PMIOPort  Port=4  Side=Right
  b : PMIOPort  Port=5  Side=Right
  c : PMIOPort  Port=6  Side=Right
  wires:
  Subsystem1/1(Out1) -> Three-Phase Breaker26/1
  [I97] -> Subsystem1/1(Iabc1)
  connections:
  VI13/LConn1 -- A/RConn1
  Three-Phase Breaker26/LConn2 -- VI13/RConn2
  Three-Phase Breaker26/LConn3 -- VI13/RConn3
  Three-Phase Breaker26/LConn1 -- VI13/RConn1
  VI13/LConn2 -- B/RConn1
  Three-Phase Breaker26/RConn1 -- a/RConn1
  VI13/LConn3 -- C/RConn1
  Three-Phase Breaker26/RConn2 -- b/RConn1
  Three-Phase Breaker26/RConn3 -- c/RConn1

== system 14_bus/Subsystem33 ==
  Subsystem1 : Subsystem
  Three-Phase Breaker26 : spsThreePhaseBreakerLib/Three-Phase Breaker  InitialState=closed  SwitchA=on  SwitchB=on  SwitchC=on  SwitchTimes="[1/60  5/60]"  External=on  BreakerResistance=0.01  SnubberResistance=1e6  SnubberCapacitance=inf  Measurements=None
  VI13 : spsThreePhaseVIMeasurementLib/Three-Phase V-I Measurement  VoltageMeasurement=no  SetLabelV=off  LabelV=Vabc  Vpu=off  VpuLL=off  CurrentMeasurement=yes  SetLabelI=on  LabelI=Ic9  Ipu=off  Pbase=100e6  Vbase=500e3  OutputType=Complex  PhasorSimulation=off  PSBequivalent=0
  A : PMIOPort  Side=Left
  B : PMIOPort  Port=2  Side=Left
  C : PMIOPort  Port=3  Side=Left
  a : PMIOPort  Port=4  Side=Right
  b : PMIOPort  Port=5  Side=Right
  c : PMIOPort  Port=6  Side=Right
  wires:
  Subsystem1/1(Out1) -> Three-Phase Breaker26/1
  [Ic9] -> Subsystem1/1(Iabc1)
  connections:
  VI13/LConn1 -- A/RConn1
  Three-Phase Breaker26/LConn2 -- VI13/RConn2
  Three-Phase Breaker26/LConn3 -- VI13/RConn3
  Three-Phase Breaker26/LConn1 -- VI13/RConn1
  VI13/LConn2 -- B/RConn1
  Three-Phase Breaker26/RConn1 -- a/RConn1
  VI13/LConn3 -- C/RConn1
  Three-Phase Breaker26/RConn2 -- b/RConn1
  Three-Phase Breaker26/RConn3 -- c/RConn1

== system 14_bus/Subsystem34 ==
  Subsystem1 : Subsystem
  Three-Phase Breaker26 : spsThreePhaseBreakerLib/Three-Phase Breaker  InitialState=closed  SwitchA=on  SwitchB=on  SwitchC=on  SwitchTimes="[1/60  5/60]"  External=on  BreakerResistance=0.01  SnubberResistance=1e6  SnubberCapacitance=inf  Measurements=None
  VI13 : spsThreePhaseVIMeasurementLib/Three-Phase V-I Measurement  VoltageMeasurement=no  SetLabelV=off  LabelV=Vabc  Vpu=off  VpuLL=off  CurrentMeasurement=yes  SetLabelI=on  LabelI=IL9  Ipu=off  Pbase=100e6  Vbase=500e3  OutputType=Complex  PhasorSimulation=off  PSBequivalent=0
  A : PMIOPort  Side=Left
  B : PMIOPort  Port=2  Side=Left
  C : PMIOPort  Port=3  Side=Left
  a : PMIOPort  Port=4  Side=Right
  b : PMIOPort  Port=5  Side=Right
  c : PMIOPort  Port=6  Side=Right
  wires:
  Subsystem1/1(Out1) -> Three-Phase Breaker26/1
  [IL9] -> Subsystem1/1(Iabc1)
  connections:
  VI13/LConn1 -- A/RConn1
  Three-Phase Breaker26/LConn2 -- VI13/RConn2
  Three-Phase Breaker26/LConn3 -- VI13/RConn3
  Three-Phase Breaker26/LConn1 -- VI13/RConn1
  VI13/LConn2 -- B/RConn1
  Three-Phase Breaker26/RConn1 -- a/RConn1
  VI13/LConn3 -- C/RConn1
  Three-Phase Breaker26/RConn2 -- b/RConn1
  Three-Phase Breaker26/RConn3 -- c/RConn1
